simulink model "pow_version_1_sim"  (R2024a)
settings: Solver=VariableStepAuto  StartTime=0.0  StopTime=T  MaxStep=sim_step  RelTol=rel_tol
values from neighbouring files (symbols this model uses):
  alpha = 0    [pow_version_1.m]
  cm = 0    [pow_version_1.m]
  d = 0    [pow_version_1.m]
  g = b    [pow_version_1.m]
  lambda0 = 0    [pow_version_1.m]
  x0 = x0_guess    [pow_version_1.m]
settings Model: Creator=elino  LastModifiedBy=elino

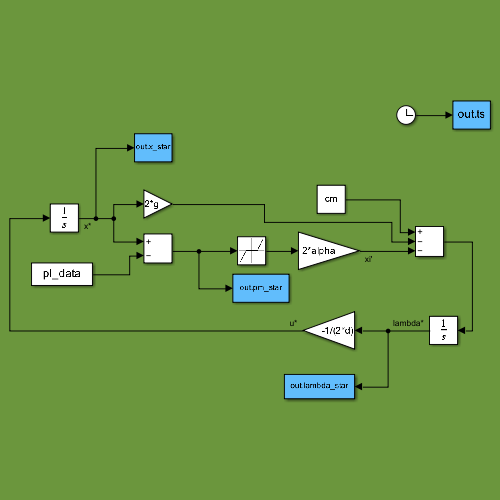
[thumbnail: Simulink's stored preview of the top-level diagram]
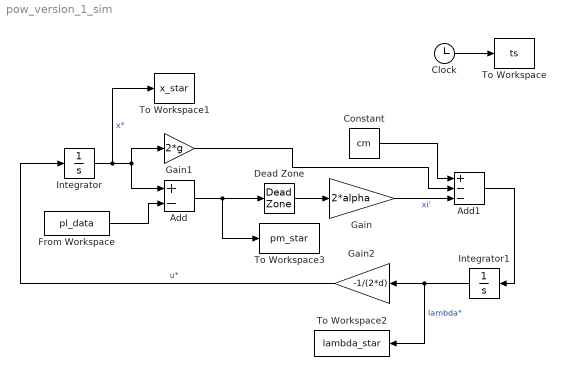
== system pow_version_1_sim ==
  Add : Sum  Inputs=+-
  Add1 : Sum  Inputs=+--
  Clock : Clock
  Constant : Constant  Value=cm
  Dead Zone : DeadZone  LowerValue=0  UpperValue=Pbar
  From Workspace : FromWorkspace  VariableName=pl_data
  Gain : Gain  Gain=2*alpha
  Gain1 : Gain  Gain=2*g
  Gain2 : Gain  Gain=-1/(2*d)
  Integrator : Integrator  InitialCondition=x0
  Integrator1 : Integrator  InitialCondition=lambda0
  To Workspace : ToWorkspace  VariableName=ts  SampleTime=-1
  To Workspace1 : ToWorkspace  VariableName=x_star  SampleTime=-1
  To Workspace2 : ToWorkspace  VariableName=lambda_star  SampleTime=-1
  To Workspace3 : ToWorkspace  VariableName=pm_star  SampleTime=-1
  wires:
  Integrator/1 -> To Workspace1/1, Gain1/1, Add/1  "x*"
  From Workspace/1 -> Add/2
  Add/1 -> To Workspace3/1, Dead Zone/1
  Dead Zone/1 -> Gain/1
  Gain/1 -> Add1/3  "xi'"
  Add1/1 -> Integrator1/1
  Gain1/1 -> Add1/2
  Constant/1 -> Add1/1
  Integrator1/1 -> To Workspace2/1, Gain2/1  "lambda*"
  Gain2/1 -> Integrator/1  "u*"
  Clock/1 -> To Workspace/1
